simulink library "INT_DReqSwt_DD"  (R2016b)
settings: Solver=VariableStepAuto  StartTime=0.0  StopTime=10.0  RelTol=1e-3
settings Model: Creator=xinchangran  LastModifiedBy=xinchangran

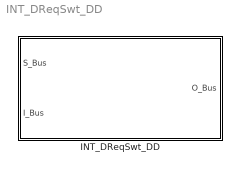
== system INT_DReqSwt_DD ==
  INT_DReqSwt_DD : Subsystem

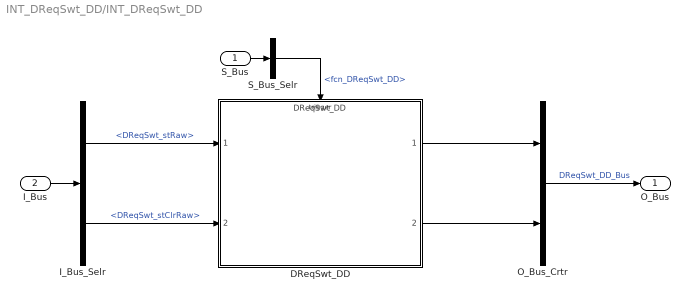
== system INT_DReqSwt_DD/INT_DReqSwt_DD ==
  S_Bus : Inport
  I_Bus : Inport  Port=2
  DReqSwt_DD : ModelReference  ModelNameDialog=DReqSwt_DD  SimulationMode=Normal  ModelReferenceVersion=1.20  TriggerPortName=function  TriggerPortTriggerType=function-call  TriggerPortStatesWhenEnabling=held
  I_Bus_Selr : BusSelector  OutputSignals=DReqSwt_stRaw,DReqSwt_stClrRaw
  O_Bus_Crtr : BusCreator  Inputs=2
  S_Bus_Selr : BusSelector  OutputSignals=fcn_DReqSwt_DD
  O_Bus : Outport
  wires:
  S_Bus_Selr/1 -> DReqSwt_DD/Trigger  "<fcn_DReqSwt_DD>"
  S_Bus/1 -> S_Bus_Selr/1
  I_Bus/1 -> I_Bus_Selr/1
  I_Bus_Selr/1 -> DReqSwt_DD/1  "<DReqSwt_stRaw>"
  I_Bus_Selr/2 -> DReqSwt_DD/2  "<DReqSwt_stClrRaw>"
  O_Bus_Crtr/1 -> O_Bus/1  "DReqSwt_DD_Bus"
  DReqSwt_DD/1 -> O_Bus_Crtr/1
  DReqSwt_DD/2 -> O_Bus_Crtr/2
